simulink model "QC_Dynamics"  (R2017b)
settings: Solver=FixedStepAuto  StartTime=0.0  StopTime=10.0  FixedStep=interval  RelTol=1e-3
values from neighbouring files (symbols this model uses):
  aefront = aetop/10    (= 0.08494)    [Sim_Constants.m]
  aeside = aetop/10    (= 0.08494)    [Sim_Constants.m]
  aetop = .8494    (= 0.8494)    [Sim_Constants.m]
  cdrag = 1.3    [Sim_Constants.m]
  dair = 1.225    [Sim_Constants.m]
  g = 9.8    [Sim_Constants.m]    (also in startup.m)
  m = 3.65    [Sim_Constants.m]    (also in startup.m)
  wb = .6    (= 0.6)    [Quad_vis.m]    (also in Sim_Constants.m; startup.m)
undefined symbols (not defined in the file or in its folder): zinitial
settings Model: Creator=DanAdmin  LastModifiedBy=DanAdmin

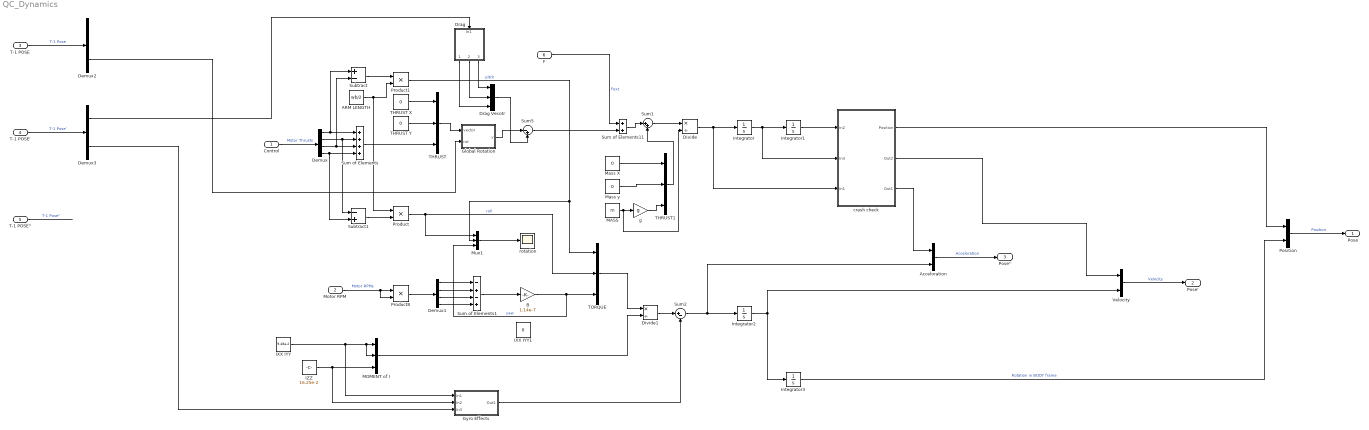
== system QC_Dynamics ==
  Control : Inport  PortDimensions=4
      settings: AttributesFormatString=4x1 vector motor thrust
  Motor RPM : Inport  Port=2  PortDimensions=4
      settings: AttributesFormatString=4x1 vector rpm
  T-1 POSE : Inport  Port=3  PortDimensions=6
      settings: AttributesFormatString=6x1 position vector. transpose([x,y,z,phi,theta,psi])
  T-1 POSE' : Inport  Port=4  PortDimensions=6
      settings: AttributesFormatString=6x1 velocity vector. transpose([x,y,z,phi,theta,psi])
  T-1 POSE'' : Inport  Port=5  PortDimensions=6
      settings: AttributesFormatString=6x1 acceloration vector. transpose([x,y,z,phi,theta,psi])
  F : Inport  Port=6  PortDimensions=3
      settings: AttributesFormatString=3x1 external force vector. transpose([x,y,z])
  ARM LENGTH : Constant  Value=wb/2
  Acceloration : Mux  Inputs=2
  B : Gain  Gain=1.14e-7
  Demux : Demux
  Demux1 : Demux
  Demux2 : Demux  Outputs=2
  Demux3 : Demux  Outputs=2
  Divide : Product  Inputs=*/
  Divide1 : Product  Inputs=*/
  Drag : Subsystem
  Drag Vecotr : Mux  Inputs=3
  Global Rotation : MATLAB Function  TreatAsAtomicUnit=on
  Gyro Effects : Subsystem
  IXX IYY : Constant  Value=9.48e-2
  IXX IYY1 : Constant  Value=0
  IZZ : Constant  Value=16.25e-2
  Integrator{,1..3} (4 alike) : Integrator
  MASS : Constant  Value=m
  MOMENT of I : Mux  Inputs=3
  Mass X : Constant  Value=0
  Mass y : Constant  Value=0
  Mux1 : Mux  Inputs=3
  Position : Mux  Inputs=2
  Product : Product
  Product1 : Product
  Product8 : Product
  Subtract : Sum  Inputs=+-
  Subtract1 : Sum  Inputs=-+
  Sum of Elements : Sum  Inputs=++++
  Sum of Elements1 : Sum  Inputs=-+-+
  Sum of Elements11 : Sum
  Sum1 : Sum  Inputs=|++
  Sum2 : Sum  Inputs=|+-
  Sum5 : Sum  Inputs=|-+
  THRUST : Mux  Inputs=3
  THRUST X : Constant  Value=0
  THRUST Y : Constant  Value=0
  THRUST1 : Mux  Inputs=3
  TORQUE : Mux  Inputs=3
  Velocity : Mux  Inputs=2
  crash check : Subsystem
  g : Gain  Gain=g
  rotation : Scope
  Pose : Outport
      settings: AttributesFormatString=6x1 true position vector, transpose([x,y,z,phi,theta,psi])
  Pose' : Outport  Port=2
      settings: AttributesFormatString=6x1 true velocity vector, transpose([x,y,z,phi,theta,psi])
  Pose'' : Outport  Port=3
      settings: AttributesFormatString=6x1 true acceloration vector, transpose([x,y,z,phi,theta,psi])
  wires:
  Demux1/3 -> Sum of Elements1/3
  F/1 -> Sum of Elements11/1  "Fext"
  Demux/2 -> Subtract1/1, Sum of Elements/2
  Velocity/1 -> Pose'/1  "Velocity"
  THRUST/1 -> Global Rotation/1(vector)
  Acceloration/1 -> Pose''/1  "Acceloration"
  Position/1 -> Pose/1  "Position"
  IXX IYY/1 -> Gyro Effects/1(In1), MOMENT of I/2, MOMENT of I/1
  Subtract1/1 -> Product/2
  Control/1 -> Demux/1  "Motor Thrusts"
  Subtract/1 -> Product1/1
  Demux1/2 -> Sum of Elements1/2
  Demux3/1 -> Drag/1(In1)
  Demux/3 -> Subtract/2, Sum of Elements/3
  MOMENT of I/1 -> Divide1/2
  Demux/4 -> Subtract1/2, Sum of Elements/4
  ARM LENGTH/1 -> Product1/2, Product/1
  Demux/1 -> Subtract/1, Sum of Elements/1
  Integrator2/1 -> Integrator3/1, Velocity/2
  MASS/1 -> g/1, Divide/2
  Sum of Elements1/1 -> B/1
  Demux3/2 -> Gyro Effects/3(In3)
  IZZ/1 -> Gyro Effects/2(In2), MOMENT of I/3
  Integrator3/1 -> Position/2  "Rotation in BODY frame"
  Motor RPM/1 -> Product8/2, Product8/1  "Motor RPMs"
  TORQUE/1 -> Divide1/1
  Demux1/1 -> Sum of Elements1/1
  Sum2/1 -> Acceloration/2, Integrator2/1
  Demux1/4 -> Sum of Elements1/4
  Demux2/2 -> Global Rotation/2(rot)
  Mass X/1 -> THRUST1/1
  Mass y/1 -> THRUST1/2
  g/1 -> THRUST1/3
  THRUST1/1 -> Sum1/2
  Sum1/1 -> Divide/1
  Global Rotation/1(y) -> Sum5/1
  Sum of Elements11/1 -> Sum1/1
  Product8/1 -> Demux1/1
  Divide1/1 -> Sum2/1
  T-1 POSE/1 -> Demux2/1  "T-1 Pose"
  T-1 POSE'/1 -> Demux3/1  "T-1 Pose'"
  T-1 POSE''/1 -> ?  "T-1 Pose''"
  THRUST X/1 -> THRUST/1
  Sum of Elements/1 -> THRUST/3
  THRUST Y/1 -> THRUST/2
  Gyro Effects/1(Out1) -> Sum2/2
  Sum5/1 -> Sum of Elements11/2
  Drag/1(Out3) -> Drag Vecotr/3
  Drag/2(Out2) -> Drag Vecotr/2
  Drag/3(Out1) -> Drag Vecotr/1
  Drag Vecotr/1 -> Sum5/2
  Integrator1/1 -> crash check/1(In2)
  crash check/3(Out1) -> Acceloration/1
  crash check/2(Out2) -> Velocity/1
  crash check/1(Position) -> Position/1
  Divide/1 -> crash check/3(In1), Integrator/1
  Integrator/1 -> crash check/2(In3), Integrator1/1
  Mux1/1 -> rotation/1
  Product1/1 -> Mux1/2, TORQUE/1  "pitch"
  Product/1 -> Mux1/1, TORQUE/2  "roll"
  B/1 -> Mux1/3, TORQUE/3  "yaw"

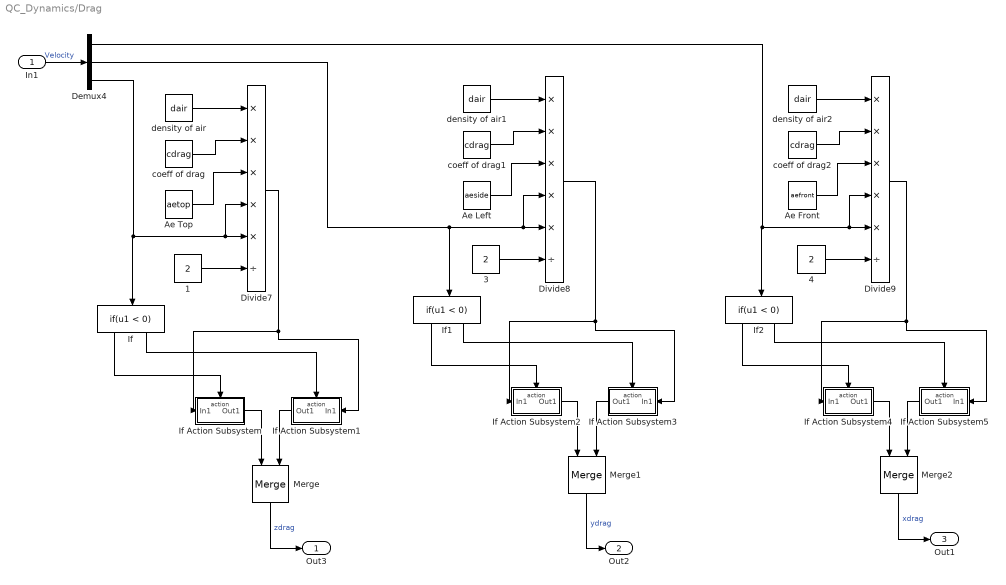
== system QC_Dynamics/Drag ==
  In1 : Inport
  1 : Constant  Value=2
  3 : Constant  Value=2
  4 : Constant  Value=2
  Ae Front : Constant  Value=aefront
  Ae Left : Constant  Value=aeside
  Ae Top : Constant  Value=aetop
  Demux4 : Demux  Outputs=3
  Divide7 : Product  Inputs=*****/
  Divide8 : Product  Inputs=*****/
  Divide9 : Product  Inputs=*****/
  If : If  IfExpression=u1 < 0
  If Action Subsystem : Subsystem  TreatAsAtomicUnit=on
  If Action Subsystem1 : Subsystem  TreatAsAtomicUnit=on
  If Action Subsystem2 : Subsystem  TreatAsAtomicUnit=on
  If Action Subsystem3 : Subsystem  TreatAsAtomicUnit=on
  If Action Subsystem4 : Subsystem  TreatAsAtomicUnit=on
  If Action Subsystem5 : Subsystem  TreatAsAtomicUnit=on
  If1 : If  IfExpression=u1 < 0
  If2 : If  IfExpression=u1 < 0
  Merge : Merge
  Merge1 : Merge
  Merge2 : Merge
  coeff of drag : Constant  Value=cdrag
  coeff of drag1 : Constant  Value=cdrag
  coeff of drag2 : Constant  Value=cdrag
  density of air : Constant  Value=dair
  density of air1 : Constant  Value=dair
  density of air2 : Constant  Value=dair
  Out3 : Outport
  Out2 : Outport  Port=2
  Out1 : Outport  Port=3
  wires:
  Demux4/3 -> Divide7/4, Divide7/5, If/1
  Demux4/1 -> If2/1, Divide9/4, Divide9/5
  coeff of drag2/1 -> Divide9/2
  4/1 -> Divide9/6
  Ae Front/1 -> Divide9/3
  density of air1/1 -> Divide8/1
  density of air2/1 -> Divide9/1
  If Action Subsystem/1(Out1) -> Merge/1
  Divide8/1 -> If Action Subsystem2/1(In1), If Action Subsystem3/1(In1)
  Merge1/1 -> Out2/1  "ydrag"
  If Action Subsystem2/1(Out1) -> Merge1/1
  If Action Subsystem3/1(Out1) -> Merge1/2
  If1/2 -> If Action Subsystem3/Action
  If1/1 -> If Action Subsystem2/Action
  Divide7/1 -> If Action Subsystem/1(In1), If Action Subsystem1/1(In1)
  Divide9/1 -> If Action Subsystem4/1(In1), If Action Subsystem5/1(In1)
  If Action Subsystem5/1(Out1) -> Merge2/2
  If2/1 -> If Action Subsystem4/Action
  If Action Subsystem4/1(Out1) -> Merge2/1
  If2/2 -> If Action Subsystem5/Action
  Merge2/1 -> Out1/1  "xdrag"
  If/2 -> If Action Subsystem1/Action
  coeff of drag1/1 -> Divide8/2
  3/1 -> Divide8/6
  Demux4/2 -> Divide8/4, Divide8/5, If1/1
  Ae Left/1 -> Divide8/3
  coeff of drag/1 -> Divide7/2
  Ae Top/1 -> Divide7/3
  1/1 -> Divide7/6
  density of air/1 -> Divide7/1
  If/1 -> If Action Subsystem/Action
  In1/1 -> Demux4/1  "Velocity"
  Merge/1 -> Out3/1  "zdrag"
  If Action Subsystem1/1(Out1) -> Merge/2

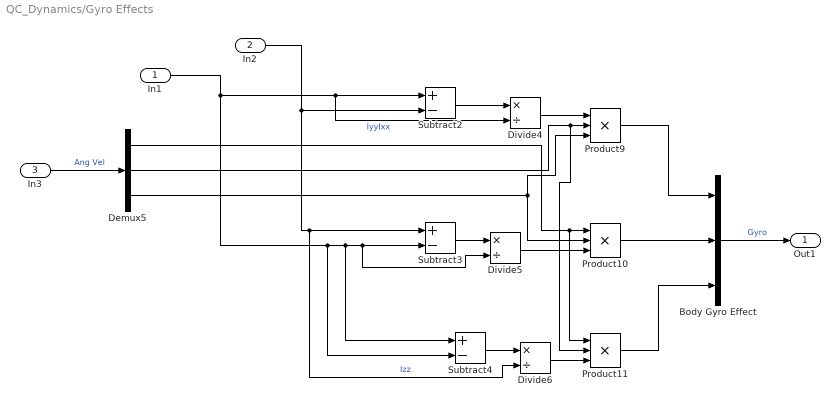
== system QC_Dynamics/Gyro Effects ==
  In1 : Inport
  In2 : Inport  Port=2
  In3 : Inport  Port=3
  Body Gyro Effect : Mux  Inputs=3
  Demux5 : Demux  Outputs=3
  Divide4 : Product  Inputs=*/
  Divide5 : Product  Inputs=*/
  Divide6 : Product  Inputs=*/
  Product10 : Product  Inputs=3
  Product11 : Product  Inputs=3
  Product9 : Product  Inputs=3
  Subtract2 : Sum  Inputs=+-
  Subtract3 : Sum  Inputs=+-
  Subtract4 : Sum  Inputs=+-
  Out1 : Outport
  wires:
  In2/1 -> Divide6/2, Subtract3/1, Subtract2/2  "Izz"
  In1/1 -> Subtract4/1, Divide5/2, Subtract3/2, Subtract4/2, Divide4/2, Subtract2/1  "IyyIxx"
  In3/1 -> Demux5/1  "Ang Vel"
  Subtract2/1 -> Divide4/1
  Divide4/1 -> Product9/1
  Demux5/2 -> Product11/2, Product9/2
  Demux5/3 -> Product9/3, Product10/2
  Divide5/1 -> Product10/3
  Product10/1 -> Body Gyro Effect/2
  Divide6/1 -> Product11/3
  Demux5/1 -> Product11/1, Product10/1
  Product11/1 -> Body Gyro Effect/3
  Subtract3/1 -> Divide5/1
  Product9/1 -> Body Gyro Effect/1
  Subtract4/1 -> Divide6/1
  Body Gyro Effect/1 -> Out1/1  "Gyro"

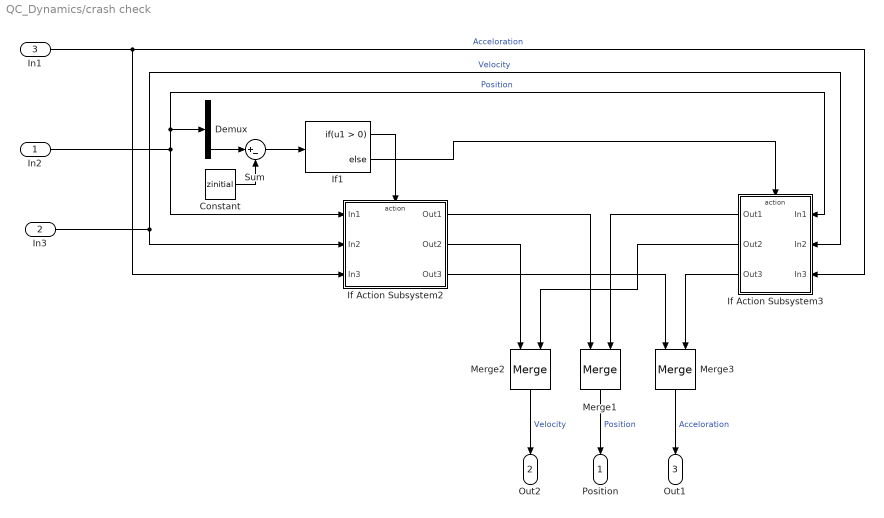
== system QC_Dynamics/crash check ==
  In2 : Inport
  In3 : Inport  Port=2
  In1 : Inport  Port=3
  Constant : Constant  Value=zinitial
  Demux : Demux  Outputs=3
  If Action Subsystem2 : Subsystem  TreatAsAtomicUnit=on
  If Action Subsystem3 : Subsystem  TreatAsAtomicUnit=on
  If1 : If
  Merge1 : Merge
  Merge2 : Merge
  Merge3 : Merge
  Sum : Sum  Inputs=|+-
  Position : Outport
  Out2 : Outport  Port=2
  Out1 : Outport  Port=3
  wires:
  Merge3/1 -> Out1/1  "Acceloration"
  If Action Subsystem3/2(Out2) -> Merge2/2
  If Action Subsystem3/3(Out3) -> Merge3/2
  If Action Subsystem2/3(Out3) -> Merge3/1
  If Action Subsystem2/2(Out2) -> Merge2/1
  In3/1 -> If Action Subsystem2/2(In2), If Action Subsystem3/2(In2)  "Velocity"
  In1/1 -> If Action Subsystem3/3(In3), If Action Subsystem2/3(In3)  "Acceloration"
  Merge2/1 -> Out2/1  "Velocity"
  If1/1 -> If Action Subsystem2/Action
  If Action Subsystem3/1(Out1) -> Merge1/2
  If Action Subsystem2/1(Out1) -> Merge1/1
  If1/2 -> If Action Subsystem3/Action
  In2/1 -> If Action Subsystem2/1(In1), Demux/1, If Action Subsystem3/1(In1)  "Position"
  Merge1/1 -> Position/1  "Position"
  Demux/3 -> Sum/1
  Constant/1 -> Sum/2
  Sum/1 -> If1/1

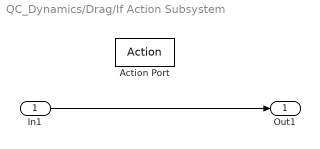
== system QC_Dynamics/Drag/If Action Subsystem ==
  In1 : Inport
  Action Port : ActionPort  ActionType=then
  Out1 : Outport
  wires:
  In1/1 -> Out1/1

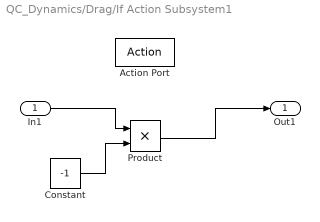
== system QC_Dynamics/Drag/If Action Subsystem1 ==
  In1 : Inport
  Action Port : ActionPort  ActionType=else
  Constant : Constant  Value=-1
  Product : Product
  Out1 : Outport
  wires:
  In1/1 -> Product/1
  Constant/1 -> Product/2
  Product/1 -> Out1/1

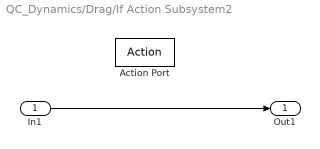
== system QC_Dynamics/Drag/If Action Subsystem2 ==
  In1 : Inport
  Action Port : ActionPort  ActionType=then
  Out1 : Outport
  wires:
  In1/1 -> Out1/1

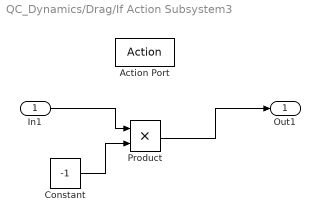
== system QC_Dynamics/Drag/If Action Subsystem3 ==
  In1 : Inport
  Action Port : ActionPort  ActionType=else
  Constant : Constant  Value=-1
  Product : Product
  Out1 : Outport
  wires:
  In1/1 -> Product/1
  Constant/1 -> Product/2
  Product/1 -> Out1/1

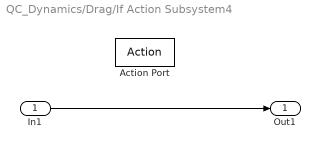
== system QC_Dynamics/Drag/If Action Subsystem4 ==
  In1 : Inport
  Action Port : ActionPort  ActionType=then
  Out1 : Outport
  wires:
  In1/1 -> Out1/1

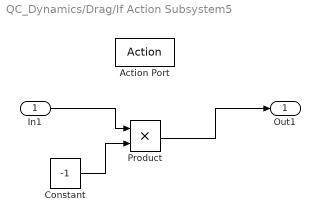
== system QC_Dynamics/Drag/If Action Subsystem5 ==
  In1 : Inport
  Action Port : ActionPort  ActionType=else
  Constant : Constant  Value=-1
  Product : Product
  Out1 : Outport
  wires:
  In1/1 -> Product/1
  Constant/1 -> Product/2
  Product/1 -> Out1/1

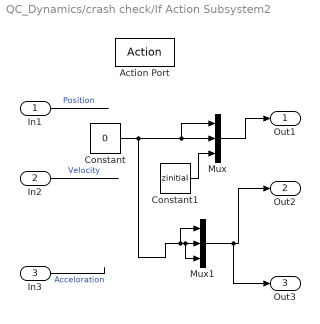
== system QC_Dynamics/crash check/If Action Subsystem2 ==
  In1 : Inport
  In2 : Inport  Port=2
  In3 : Inport  Port=3
  Action Port : ActionPort  ActionType=then
  Constant : Constant  Value=0
  Constant1 : Constant  Value=zinitial
  Mux : Mux  Inputs=3
  Mux1 : Mux  Inputs=3
  Out1 : Outport  InitialOutput=[0]
  Out2 : Outport  Port=2  InitialOutput=[0]
  Out3 : Outport  Port=3  InitialOutput=[0]
  wires:
  In1/1 -> ?  "Position"
  In2/1 -> ?  "Velocity"
  In3/1 -> ?  "Acceloration"
  Constant/1 -> Mux/2, Mux/1, Mux1/1, Mux1/3, Mux1/2
  Mux/1 -> Out1/1
  Constant1/1 -> Mux/3
  Mux1/1 -> Out3/1, Out2/1

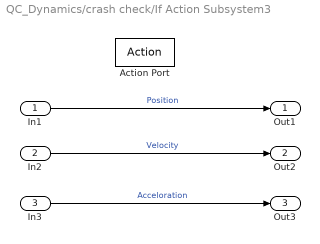
== system QC_Dynamics/crash check/If Action Subsystem3 ==
  In1 : Inport
  In2 : Inport  Port=2
  In3 : Inport  Port=3
  Action Port : ActionPort  ActionType=else
  Out1 : Outport
  Out2 : Outport  Port=2
  Out3 : Outport  Port=3
  wires:
  In1/1 -> Out1/1  "Position"
  In2/1 -> Out2/1  "Velocity"
  In3/1 -> Out3/1  "Acceloration"

== matlab function QC_Dynamics/Global Rotation ==
  data: vector input size=[3 1]; y output size=[3 1]; rot input size=[3 1]
function y = fcn(vector, rot)


%R=[1,0,0;0,cos(rot(1)),-sin(rot(1));0,sin(rot(1)),cos(rot(1))]*[cos(rot(2)),0, -sin(rot(2));0,1,0;sin(rot(2)),0,cos(rot(2))]*[cos(rot(3)),-sin(rot(3)),0;sin(rot(3)),cos(rot(3)),0;0,0,1];

Rx=[1,0,0;0,cos(rot(1)),-sin(rot(1));0,sin(rot(1)),cos(rot(1))];
%Ry=[cos(rot(2)),-sin(rot(2)),0;sin(rot(2)),cos(rot(2)),0;0,0,1];
Ry=[cos(rot(2)),0, sin(rot(2));0,1,0;-sin(rot(2)),0,cos(rot(2))];
Rz=[cos(rot(3)),-sin(rot(3)),0;sin(rot(3)),cos(rot(3)),0;0,0,1];

R=Rz*Ry*Rx;


w=R*vector;
y=w;
end
